simulink model "guid_stab_loop_no_rot"  (R2021a)
settings: Solver=VariableStepAuto  StartTime=0.0  StopTime=20  RelTol=1e-3
settings Model: Creator=AutomZ2-RG02A02  LastModifiedBy=AutomZ2-RG02A02

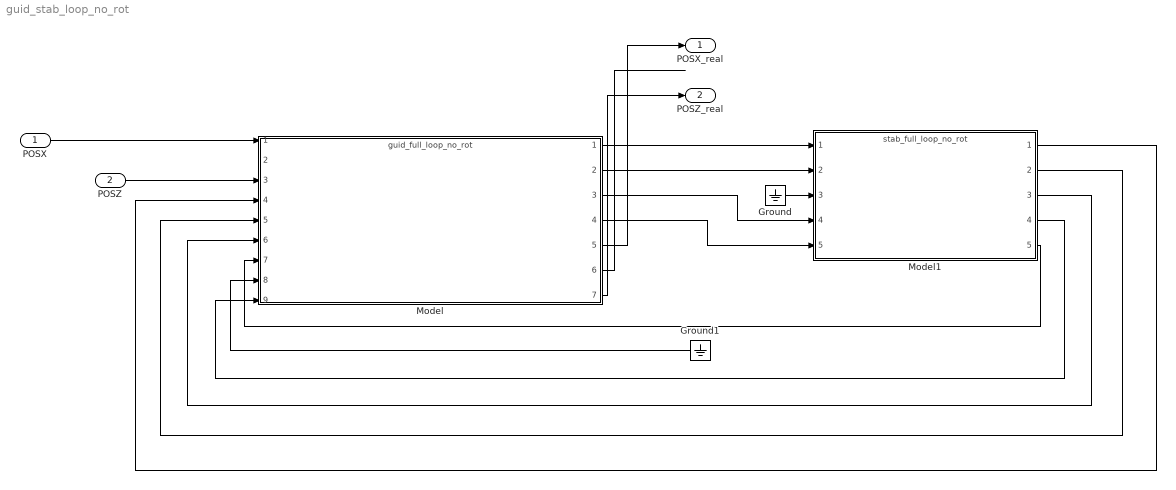
== system guid_stab_loop_no_rot ==
  POSX : Inport
  POSZ : Inport  Port=2
  Ground : Ground
  Ground1 : Ground
  Model : ModelReference  ModelNameDialog=guid_full_loop_no_rot.slx  SimulationMode=Normal  ModelReferenceVersion=72
  Model1 : ModelReference  ModelNameDialog=stab_full_loop_no_rot.slx  SimulationMode=Normal  ModelReferenceVersion=63
  POSX_real : Outport
  POSZ_real : Outport  Port=2
  wires:
  Model/1 -> Model1/1
  Model/2 -> Model1/2
  Model/3 -> Model1/4
  Model/4 -> Model1/5
  Ground/1 -> Model1/3
  Model1/1 -> Model/4
  Model1/2 -> Model/5
  Model1/3 -> Model/6
  Model1/5 -> Model/7
  Ground1/1 -> Model/8
  Model1/4 -> Model/9
  POSZ/1 -> Model/3
  POSX/1 -> Model/1
  ? -> Model/2
  Model/5 -> POSX_real/1
  Model/6 -> ?
  Model/7 -> POSZ_real/1
